simulink library "apparentWind_ul"  (R2022a)
settings: Solver=VariableStepAuto  StartTime=0.0  StopTime=10.0  RelTol=1e-3
settings Model: Creator=mcobb  LastModifiedBy=lhill8
settings SolverCC: AlgebraicLoopSolver=TrustRegion
settings DebuggingCC: UnconnectedInputMsg=warning  UnconnectedOutputMsg=warning  UnconnectedLineMsg=warning  SFMachineParentedDataDiag=warning  ArithmeticOperatorsInVariantConditions=warning
settings SFSimCC: CustomCodeUndefinedFunction=UseInterfaceOnly

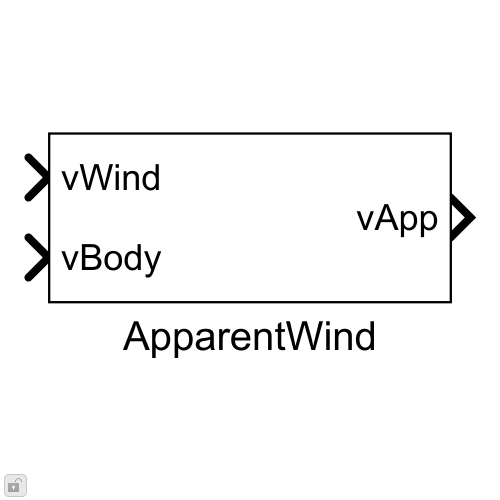
[thumbnail: Simulink's stored preview of the top-level diagram]
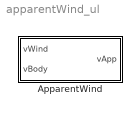
== system apparentWind_ul ==
  ApparentWind : Subsystem

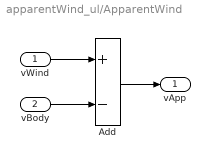
== system apparentWind_ul/ApparentWind ==
  vWind : Inport
  vBody : Inport  Port=2
  Add : Sum  Inputs=+-
  vApp : Outport  VectorParamsAs1DForOutWhenUnconnected=off
  wires:
  vBody/1 -> Add/2
  vWind/1 -> Add/1
  Add/1 -> vApp/1
